simulink model "continuous_observed_controller_emc"  (R2022a)
settings: Solver=ode45  StartTime=0.0  StopTime=100  RelTol=1e-3
values from neighbouring files (symbols this model uses):
  A = [0 0 1 0 0 ... (first row only)    [DesignProjectP2.m]    (also in DesignProjectP3.m; DesignProject_OffsetP3.m; mpc_example_regulation.m = [ 	 0,       0,              1,  0, 0; 	 0,       0,        ; mpc_example_tracking.m = [ 	 0,       0,              1,  0, 0; 	 0,       0,        )
  B = [0;0;0;0;1/La]    [DesignProjectP2.m]    (also in DesignProjectP3.m; DesignProject_OffsetP3.m; mpc_example_regulation.m = [0; 0; 0; 0; 1/La]; mpc_example_tracking.m = [0; 0; 0; 0; 1/La])
  C = [1 0 0 0 0 ... (first row only)    [DesignProjectP2.m]    (also in DesignProjectP3.m; DesignProject_OffsetP3.m; mpc_example_regulation.m; mpc_example_tracking.m)
  init = [theta_m_init; theta_l_init; thetadot_m_init; thetadot_l_init; Ia_init]    [ELEN90064_Project_Parameters.m]
  K_cont = Kcont(2:6)    [phase2_emc.m]
  Ki_cont = Kcont(1)    [phase2_emc.m]
  L = place(A', C', observer_poles)'    [DesignProjectP2.m]    (also in DesignProjectP3.m; DesignProject_OffsetP3.m = L_t'; phase2_emc.m = place(A',C',desired_obsv_poles)')
settings Model: Creator=Einon  LastModifiedBy=Einon

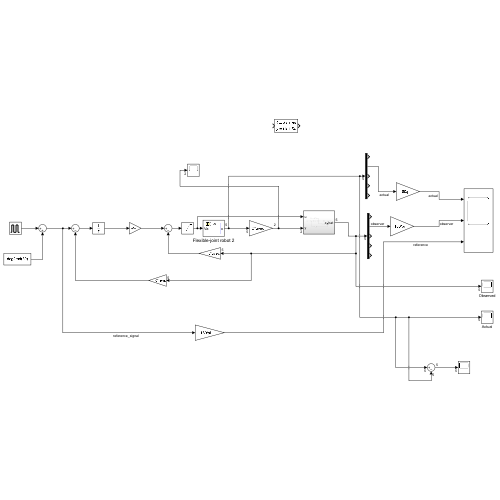
[thumbnail: Simulink's stored preview of the top-level diagram]
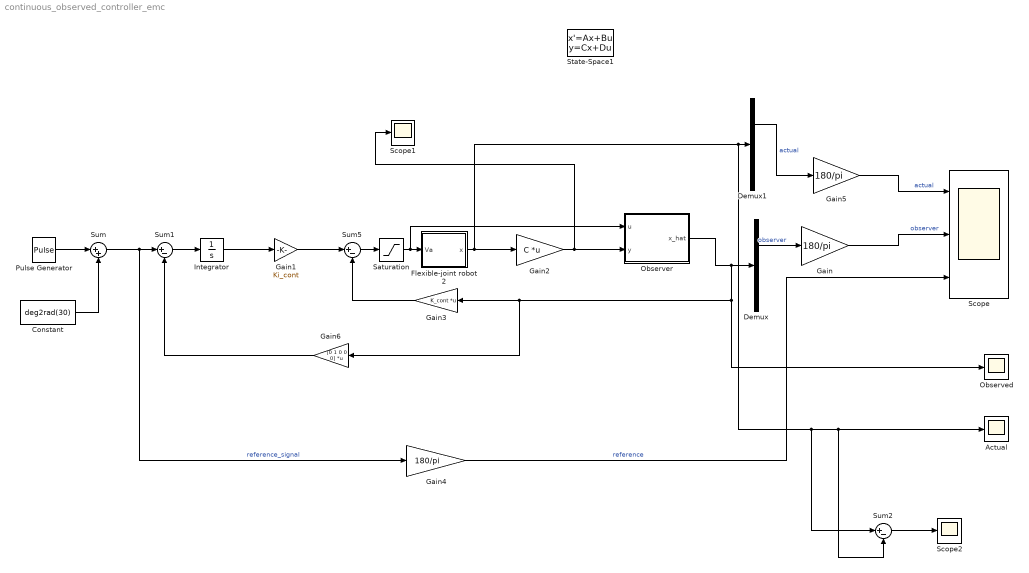
== system continuous_observed_controller_emc ==
  Actual : Scope
  Constant : Constant  Value=deg2rad(30)
  Demux : Demux  Outputs=5
  Demux1 : Demux  Outputs=5
  Flexible-joint robot 2 : Subsystem
      mask Display: image('$imagefile'); % Use "Edit Image" on toolstrip to change.
  Gain : Gain  Gain=180/pi
  Gain1 : Gain  Gain=Ki_cont
  Gain2 : Gain  Gain=C  Multiplication=Matrix(K*u) (u vector)
  Gain3 : Gain  Gain=K_cont  Multiplication=Matrix(K*u) (u vector)
  Gain4 : Gain  Gain=180/pi
  Gain5 : Gain  Gain=180/pi
  Gain6 : Gain  Gain=[0 1 0 0 0]  Multiplication=Matrix(K*u) (u vector)
  Integrator : Integrator
  Observed : Scope
  Observer : Subsystem
  Pulse Generator : DiscretePulseGenerator  PulseType=Time based  Amplitude=deg2rad(30)  Period=40  PulseWidth=50
  Saturation : Saturate  UpperLimit=6  LowerLimit=-6
  Scope : Scope  NumInputPorts=3
  Scope1 : Scope
  Scope2 : Scope
  State-Space1 : StateSpace  A=A  B=B  C=eye(5)  D=zeros(5,1)  InitialCondition=init
  Sum : Sum  Inputs=|++
  Sum1 : Sum  Inputs=|+-
  Sum2 : Sum  Inputs=|+-
  Sum5 : Sum  Inputs=|+-
  wires:
  Sum/1 -> Sum1/1, Gain4/1  "reference_signal"
  Gain3/1 -> Sum5/2
  Flexible-joint robot 2/1(x) -> Sum2/1, Sum2/2, Actual/1, Demux1/1, Gain2/1
  Gain2/1 -> Scope1/1, Observer/2(y)
  Observer/1(x_hat) -> Observed/1, Gain6/1, Gain3/1, Demux/1
  Demux/2 -> Gain/1  "observer"
  Demux1/2 -> Gain5/1  "actual"
  Gain4/1 -> Scope/3  "reference"
  Gain/1 -> Scope/2  "observer"
  Gain5/1 -> Scope/1  "actual"
  Integrator/1 -> Gain1/1
  Gain1/1 -> Sum5/1
  Pulse Generator/1 -> Sum/1
  Constant/1 -> Sum/2
  Sum1/1 -> Integrator/1
  Gain6/1 -> Sum1/2
  Sum2/1 -> Scope2/1
  Sum5/1 -> Saturation/1
  Saturation/1 -> Observer/1(u), Flexible-joint robot 2/1(Va)

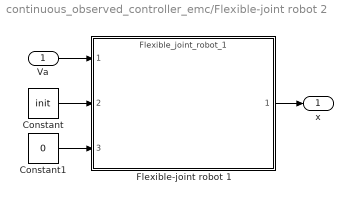
== system continuous_observed_controller_emc/Flexible-joint robot 2 ==
  Va : Inport
  Constant : Constant  Value=init
  Constant1 : Constant  Value=0
  Flexible-joint robot 1 : ModelReference  ModelNameDialog=Flexible_joint_robot_1  ModelReferenceVersion=1.65  CopyOfModelProtected=on
  x : Outport
  wires:
  Constant/1 -> Flexible-joint robot 1/2
  Constant1/1 -> Flexible-joint robot 1/3
  Flexible-joint robot 1/1 -> x/1
  Va/1 -> Flexible-joint robot 1/1

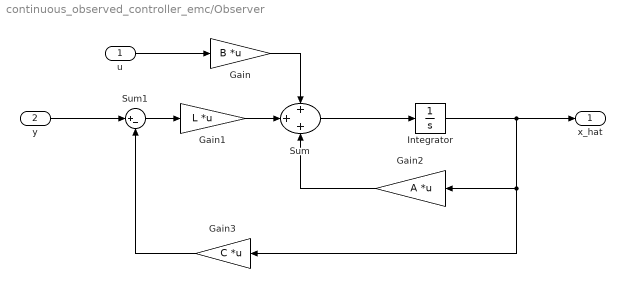
== system continuous_observed_controller_emc/Observer ==
  u : Inport
  y : Inport  Port=2  OutDataTypeStr=double
  Gain : Gain  Gain=B  Multiplication=Matrix(K*u) (u vector)
  Gain1 : Gain  Gain=L  Multiplication=Matrix(K*u) (u vector)
  Gain2 : Gain  Gain=A  Multiplication=Matrix(K*u) (u vector)
  Gain3 : Gain  Gain=C  Multiplication=Matrix(K*u) (u vector)
  Integrator : Integrator
  Sum : Sum  Inputs=+++
  Sum1 : Sum  Inputs=|+-
  x_hat : Outport
  wires:
  u/1 -> Gain/1
  Gain/1 -> Sum/1
  y/1 -> Sum1/1
  Sum1/1 -> Gain1/1
  Sum/1 -> Integrator/1
  Integrator/1 -> x_hat/1, Gain3/1, Gain2/1
  Gain3/1 -> Sum1/2
  Gain2/1 -> Sum/3
  Gain1/1 -> Sum/2
